simulink model "GammaCorrection_base"  (R2016a)
settings: Solver=VariableStepAuto  StartTime=0.0  StopTime=inf  RelTol=1e-3
undefined symbols (not defined in the file): gray
libraries: ModelComposer x6, visionsinks x2, dspvision x1
settings Model: Creator=ukumar  LastModifiedBy=wesleyl

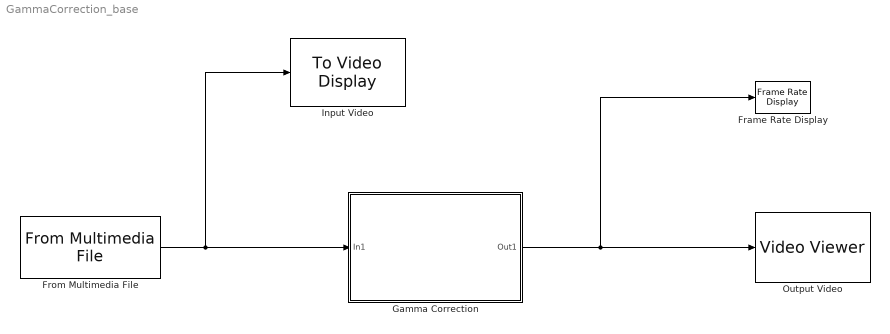
== system GammaCorrection_base ==
  Frame Rate Display : visionsinks/Frame Rate Display  UpdateRate=10
  From Multimedia File : dspvision/From Multimedia File  inputFilename=handshake_left.avi  loop=on  numPlays=inf  outputStreams=Video only  videoDataType=uint8  audioDataType=int16  inheritSampleTime=off  userDefinedSampleTime=1/30  noAudioOutput=off  isIntensityVideo=off  fourcc=Intensity  colorVideoFormat=One multidimensional signal  outputEOF=off  dataOrg=Column-major  audioFrameSize=1024  computeAudioFrameSize=off  outSamplingMode=Sample based
  Gamma Correction : Subsystem
  Input Video : visionsinks/To Video Display  windowSizeMode=True size (1:1)  openAtMdlStart=on  fullScreen=off  videoWindowX=536805376  videoWindowY=536805376  saveWindowSize=off  videoWindowWidth=2147483647  videoWindowHeight=2147483647  inputColorFormat=RGB  inputType=Obsolete  imagePorts=One multidimensional signal  OutputDevice=On-screen video monitor  dataOrg=Column-major  isWindowOpen=off
  Output Video : VideoViewer  colormapValue=gray(256)  FigPos=[365 726.8 614.4 360]
  wires:
  From Multimedia File/1 -> Input Video/1, Gamma Correction/1(In1)
  Gamma Correction/1(Out1) -> Output Video/1, Frame Rate Display/1

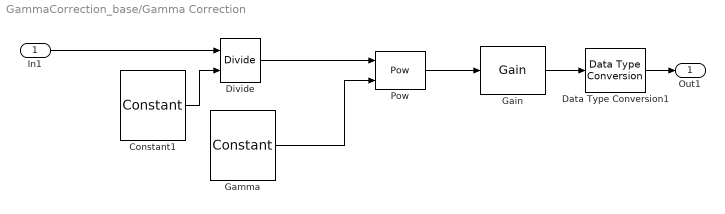
== system GammaCorrection_base/Gamma Correction ==
  In1 : Inport
  Constant1 : ModelComposer/Constant  Description=Performs multiplication  Value=255  SampleTime=-1  OutDataType=single  TypeExp=''  Signedness=Signed  WordLength=16  FractionalLength=10  RoundingMode=Truncation to minus infinity  OverflowMode=Wrap around
  Data Type Conversion1 : ModelComposer/Data Type Conversion  OutDataType=uint8  TypeExp=''  Signedness=Signed  WordLength=16  FractionalLength=10  RoundingMode=Truncation to minus infinity  OverflowMode=Wrap around
  Divide : ModelComposer/Divide  Description=Performs multiplication
  Gain : ModelComposer/Gain  Description=Performs multiplication  Gain=255  OutDataType=uint8  TypeExp=''  Signedness=Signed  WordLength=16  FractionalLength=10  RoundingMode=Truncation to minus infinity  OverflowMode=Wrap around  OutputTypeAsInput=off
  Gamma : ModelComposer/Constant  Description=Performs multiplication  Value=0.45  SampleTime=-1  OutDataType=single  TypeExp=''  Signedness=Signed  WordLength=16  FractionalLength=10  RoundingMode=Truncation to minus infinity  OverflowMode=Wrap around
  Pow : ModelComposer/Pow  Description=Performs multiplication
  Out1 : Outport
  wires:
  Gain/1 -> Data Type Conversion1/1
  Pow/1 -> Gain/1
  Gamma/1 -> Pow/2
  Data Type Conversion1/1 -> Out1/1
  Constant1/1 -> Divide/2
  Divide/1 -> Pow/1
  In1/1 -> Divide/1
